simulink model "Power_Model_Official_Pars_2022a"  (R2022a)
settings: Solver=ode23t  StartTime=0.0  StopTime=500  RelTol=1e-3
values from neighbouring files (symbols this model uses):
  anode_tube_D = 0.01    [fuel_cell_battery_par.mat]
  cathode_tube_D = 0.05    [fuel_cell_battery_par.mat]
  comp_rpm_TLU = [0 1800 3600]    [fuel_cell_battery_par.mat]
  coolant_num_layers = 20    [fuel_cell_battery_par.mat]
  coolant_num_passes = 12    [fuel_cell_battery_par.mat]
  coolant_tube_D = 0.05    [fuel_cell_battery_par.mat]
  coolant_w_channels = 1    [fuel_cell_battery_par.mat]
  env_p = 0.101325    [fuel_cell_battery_par.mat]
  env_T = 20    [fuel_cell_battery_par.mat]
  env_yH20 = 0.0115436377169    [fuel_cell_battery_par.mat]
  env_yO2 = 0.21    [fuel_cell_battery_par.mat]
  radiator_air_area_fins = 11.5625    [fuel_cell_battery_par.mat]
  radiator_air_area_primary = 1.223125    [fuel_cell_battery_par.mat]
  radiator_eta_fin = 0.7    [fuel_cell_battery_par.mat]
  radiator_N_tubes = 25    [fuel_cell_battery_par.mat]
  radiator_rho = 2700    [fuel_cell_battery_par.mat]
  radiator_t_wall = 0.0001    [fuel_cell_battery_par.mat]
  radiator_tube_H = 0.0015    [fuel_cell_battery_par.mat]
  radiator_W = 0.025    [fuel_cell_battery_par.mat]
  stack_area = 280    [fuel_cell_battery_par.mat]
  stack_iL = 1.4    [fuel_cell_battery_par.mat]
  stack_mea_rho = 1800    [fuel_cell_battery_par.mat]
  stack_num_cells = 400    [fuel_cell_battery_par.mat]
  stack_num_channels = 8    [fuel_cell_battery_par.mat]
  stack_t_gdl = 250    [fuel_cell_battery_par.mat]
  stack_t_membrane = 125    [fuel_cell_battery_par.mat]
  stack_w_channels = 1    [fuel_cell_battery_par.mat]
undefined symbols (not defined in the file or in its folder): Bat, BattCapInit, BattChargeMax, BattTempBp, CapLUTBp, CapSOCBp, Em, f_fc_auxpower, f_fc_currcmd_bpt, f_fc_h2flow, f_fc_heatflow, f_fc_tmpcmd_bpt, f_fc_voltage, Mot, Np, Ns, RInt, Tc_Batt
libraries: fl_lib x89, nesl_utility x39, FuelCell_lib x32, ee_lib x3, slpidlib x3, batteryecm_lib x1, simulink_extras x1, autolibshared x1, simulink x1
(part 3 of 4)

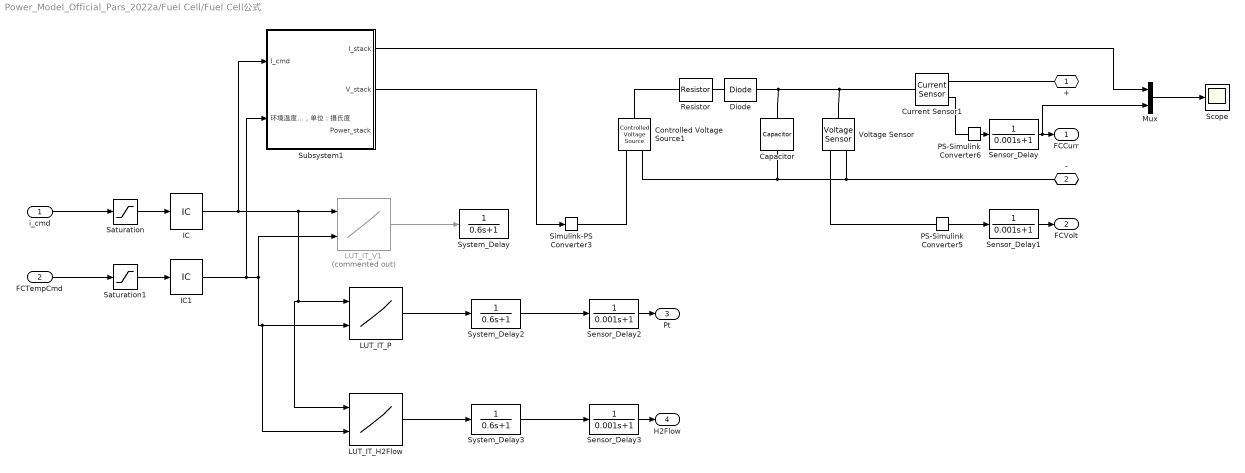
== system Power_Model_Official_Pars_2022a/Fuel Cell/Fuel Cell/公式 ==
  i_cmd : Inport
  FCTempCmd : Inport  Port=2
  Capacitor : fl_lib/Electrical/Electrical Elements/Capacitor  c=1e-6 F  r=1e-6 Ohm  g=0 1/Ohm  i_specify=off  i_priority=None  i=0 A  i_nominal_specify=off  i_nominal_unit=A  i_nominal_value=1  v_specify=off  v_priority=None  v=0 V  v_nominal_specify=off  v_nominal_unit=V  v_nominal_value=1  vc_specify=on  vc_priority=High  vc=f_fc_voltage(1) V  vc_nominal_specify=off  vc_nominal_unit=V  vc_nominal_value=1
  Controlled Voltage Source1 : fl_lib/Electrical/Electrical Sources/Controlled Voltage Source
  Current Sensor1 : fl_lib/Electrical/Electrical Sensors/Current Sensor
  Diode : fl_lib/Electrical/Electrical Elements/Diode  Vf=0.6 V  Ron=0.3 Ohm  Goff=1e-8 1/Ohm  i_specify=off  i_priority=None  i=0 A  i_nominal_specify=off  i_nominal_unit=A  i_nominal_value=1  v_specify=off  v_priority=None  v=0 V  v_nominal_specify=off  v_nominal_unit=V  v_nominal_value=1
  IC : InitialCondition  Value=f_fc_currcmd_bpt(1)
  IC1 : InitialCondition  Value=f_fc_tmpcmd_bpt(1)
  LUT_IT_H2Flow : Lookup_n-D  BreakpointsForDimension1=f_fc_currcmd_bpt  BreakpointsForDimension2=f_fc_tmpcmd_bpt  Table=f_fc_h2flow  InternalRulePriority=Speed  RndMeth=Simplest
      settings: InputPortMap=u0,u1
  LUT_IT_P : Lookup_n-D  BreakpointsForDimension1=f_fc_currcmd_bpt  BreakpointsForDimension2=f_fc_tmpcmd_bpt  Table=f_fc_auxpower  InternalRulePriority=Speed  RndMeth=Simplest
      settings: InputPortMap=u0,u1
  LUT_IT_V1 : Lookup_n-D  Commented=on  BreakpointsForDimension1=f_fc_currcmd_bpt  BreakpointsForDimension2=f_fc_tmpcmd_bpt  Table=f_fc_voltage  InternalRulePriority=Speed  RndMeth=Simplest
      settings: InputPortMap=u0,u1
  Mux : Mux  Inputs=2
  PS-Simulink Converter5 : nesl_utility/PS-Simulink Converter  PhysicalDomain=network_engine_domain  SubClassName=ps_output  LeftPortType=input  RightPortType=output  PseudoPeriodic=off  Frequencies=[]  VectorFormat=1-D array  Unit=inherit  AffineConversion=off
  PS-Simulink Converter6 : nesl_utility/PS-Simulink Converter  PhysicalDomain=network_engine_domain  SubClassName=ps_output  LeftPortType=input  RightPortType=output  PseudoPeriodic=off  Frequencies=[]  VectorFormat=1-D array  Unit=1  AffineConversion=off
  Resistor : fl_lib/Electrical/Electrical Elements/Resistor  R=1e-3 Ohm  i_specify=off  i_priority=None  i=0 A  i_nominal_specify=off  i_nominal_unit=A  i_nominal_value=1  v_specify=off  v_priority=None  v=0 V  v_nominal_specify=off  v_nominal_unit=V  v_nominal_value=1
  Saturation : Saturate  UpperLimit=max(f_fc_currcmd_bpt)  LowerLimit=0
  Saturation1 : Saturate  UpperLimit=max(f_fc_tmpcmd_bpt)  LowerLimit=0
  Scope : Scope
  Sensor_Delay{,1..3} (4 alike) : TransferFcn  Denominator=[0.001 1]
  Simulink-PS Converter3 : nesl_utility/Simulink-PS Converter  PhysicalDomain=network_engine_domain  SubClassName=ps_input  LeftPortType=input  RightPortType=output  PseudoPeriodic=off  Frequencies=[]  NoiseDistribution=none  NoiseParameters=[]  Unit=V  AffineConversion=off  FilteringAndDerivatives=provide  SimscapeFilterOrder=1  InputFilterTimeConstant=0.001  UdotUserProvided=0
  Subsystem1 : Subsystem
  System_Delay : TransferFcn  Denominator=[0.6 1]
  System_Delay2 : TransferFcn  Denominator=[0.6 1]
  System_Delay3 : TransferFcn  Denominator=[0.6 1]
  Voltage Sensor : fl_lib/Electrical/Electrical Sensors/Voltage Sensor
  + : PMIOPort  Side=Right
  - : PMIOPort  Port=2  Side=Right
  FCCurr : Outport
  FCVolt : Outport  Port=2
  Pt : Outport  Port=3
  H2Flow : Outport  Port=4
  wires:
  LUT_IT_H2Flow/1 -> System_Delay3/1
  System_Delay3/1 -> Sensor_Delay3/1
  Saturation1/1 -> IC1/1
  LUT_IT_V1/1 -> System_Delay/1
  Sensor_Delay/1 -> Mux/2, FCCurr/1
  IC1/1 -> Subsystem1/2(环境温度：T，单位：摄氏度), LUT_IT_V1/2, LUT_IT_H2Flow/2, LUT_IT_P/2
  Saturation/1 -> IC/1
  LUT_IT_P/1 -> System_Delay2/1
  IC/1 -> Subsystem1/1(I_cmd), LUT_IT_H2Flow/1, LUT_IT_P/1, LUT_IT_V1/1
  FCTempCmd/1 -> Saturation1/1
  i_cmd/1 -> Saturation/1
  Sensor_Delay2/1 -> Pt/1
  Sensor_Delay3/1 -> H2Flow/1
  PS-Simulink Converter5/1 -> Sensor_Delay1/1
  Sensor_Delay1/1 -> FCVolt/1
  PS-Simulink Converter6/1 -> Sensor_Delay/1
  Subsystem1/2(V_stack) -> Simulink-PS Converter3/1
  System_Delay2/1 -> Sensor_Delay2/1
  Subsystem1/1(I_stack) -> Mux/1
  Mux/1 -> Scope/1
  connections:
  Capacitor/RConn1 -- Voltage Sensor/RConn2 -- -/RConn1 -- Controlled Voltage Source1/RConn2
  Capacitor/LConn1 -- Diode/RConn1 -- Voltage Sensor/LConn1 -- Current Sensor1/LConn1
  +/RConn1 -- Current Sensor1/RConn2
  PS-Simulink Converter5/LConn1 -- Voltage Sensor/RConn1
  PS-Simulink Converter6/LConn1 -- Current Sensor1/RConn1
  Simulink-PS Converter3/RConn1 -- Controlled Voltage Source1/RConn1
  Resistor/RConn1 -- Diode/LConn1
  Resistor/LConn1 -- Controlled Voltage Source1/LConn1

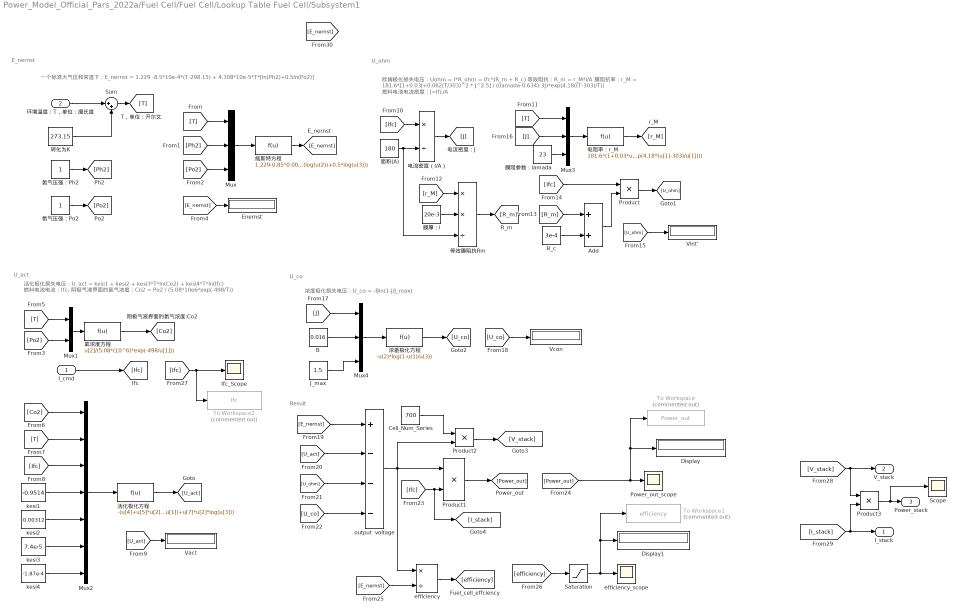
== system Power_Model_Official_Pars_2022a/Fuel Cell/Fuel Cell/Lookup Table Fuel Cell/Subsystem1 ==
  note: Result
  note: U_co
  note: 浓度极化损失电压：U_co = -Bln(1-J/J_max)
  note: U_ohm
  note: 欧姆极化损失电压：Uohm = I*R_ohm = Ifc*(R_m + R_c)
      | 等效阻抗：R_m = r_M*l/A
      | 膜阻抗率：r_M = 181.6*[1+0.03J+0.062(T/303)^2 * J^2.5] / ((lamada-0.634)-3J)*exp(4.18((T-303)/T))
      | 燃料电池电流密度：J=Ifc/A
  note: U_act
  note: 活化极化损失电压：U_act = kesi1 + kesi2 + kesi3*T*ln(Co2) + kesi4*T*ln(Ifc)
      | 燃料电池电流：Ifc;
      | 阴极气液界面的氧气浓度：Co2 = Po2 / (5.08*10e6*exp(-498/T))
  note: E_nernst
  note: 一个标准大气压和常温下：E_nernst = 1.229 -8.5*10e-4*(T-298.15) + 4.308*10e-5*T*[ln(Ph2)+0.5ln(Po2)]
  I_cmd : Inport
  环境温度：T，单位：摄氏度 : Inport  Port=2
  Add : Sum
  B : Constant  Value=0.016
  Cell_Num_Series : Constant  Value=700
  Display : Display
  Display1 : Display
  Enernst : Display
      settings: Decimation=5
  Ifc_Scope : Scope
  J_max : Constant  Value=1.5
  Mux : Mux  Inputs=3
  Mux1 : Mux  Inputs=2
  Mux2 : Mux  Inputs=7
  Mux3 : Mux  Inputs=3
  Mux4 : Mux  Inputs=3
  Power_out_scope : Scope
  Product{,1..3} (4 alike) : Product
  R_c : Constant  Value=3e-4
  Saturation : Saturate  UpperLimit=0.9  LowerLimit=0
  Scope : Scope
  Sum : Sum  Inputs=|++
  To Workspace : ToWorkspace  Commented=on  VariableName=Power_out  SampleTime=-1
      settings: Save2DSignal=2-D array (concatenate along first dimension)
  To Workspace1 : ToWorkspace  Commented=on  VariableName=efficiency  SampleTime=-1
      settings: Save2DSignal=2-D array (concatenate along first dimension)
  To Workspace2 : ToWorkspace  Commented=on  VariableName=Ifc  SampleTime=-1
      settings: Save2DSignal=2-D array (concatenate along first dimension)
  Vact : Display
      settings: Decimation=5
  Vcon : Display
      settings: Decimation=5
  Vint' : Display
      settings: Decimation=5
  efficiency : Product  Inputs=*/  OutDataTypeStr=double
  efficiency_scope : Scope
  kesi1 : Constant  Value=-0.9514
  kesi2 : Constant  Value=0.00312
  kesi3 : Constant  Value=7.4e-5
  kesi4 : Constant  Value=-1.87e-4
  output  voltage : Sum  Inputs=+---  OutDataTypeStr=double
  氢气压强：Ph2 : Constant
  氧气压强：Po2 : Constant
  氧浓度方程 : Fcn  Expr=u[2]/(5.08*(10^6)*exp(-498/u[1]))
  活化极化方程 : Fcn  Expr=-(u[4]+u[5]*u[2]+u[6]*u[2]*log(u[1])+u[7]*u[2]*log(u[3]))
  浓差极化方程 : Fcn  Expr=-u(2)*log(1-u(1)/u(3))
  电流密度（I/A） : Product  Inputs=*/  OutDataTypeStr=double
  电阻率：r_M : Fcn  Expr=181.6*(1+0.03*u[2]+0.062*((u[1]/303)^2)*(u[2]^2.5))/((u[3]-0.634-3*u[2])*(exp(4.18*(u[1]-303)/u[1])))
  等效膜阻抗Rm : Product  Inputs=**/  OutDataTypeStr=double
  能斯特方程 : Fcn  Expr=1.229-0.85*0.001*(u(1)-298.15)+4.3085*0.00001*u(1)*(log(u(2))+0.5*log(u(3)))
  膜厚：l : Constant  Value=20e-3
  膜阻参数：lamada : Constant  Value=23
  转化为K : Constant  Value=273.15
  面积(A) : Constant  Value=180
  I_stack : Outport
  V_stack : Outport  Port=2
  Power_stack : Outport  Port=3
  wires:
  [E_nernst] -> efficiency/2
  环境温度：T，单位：摄氏度/1 -> Sum/1
  [T] -> Mux/1
  Sum/1 -> [T]
  [Ifc] -> 电流密度（I/A）/1
  [Co2] -> Mux2/1
  Mux2/1 -> 活化极化方程/1
  [T] -> Mux2/2
  转化为K/1 -> Sum/2
  能斯特方程/1 -> [E_nernst]
  [Ifc] -> To Workspace2/1, Ifc_Scope/1
  Saturation/1 -> efficiency_scope/1, To Workspace1/1, Display1/1
  面积(A)/1 -> 电流密度（I/A）/2, 等效膜阻抗Rm/3
  [T] -> Mux1/1
  活化极化方程/1 -> [U_act]
  电流密度（I/A）/1 -> [J]
  output  voltage/1 -> Product2/2, efficiency/1, Product1/1
  [U_act] -> output  voltage/2
  氧气压强：Po2/1 -> [Po2]
  [r_M] -> 等效膜阻抗Rm/1
  氢气压强：Ph2/1 -> [Ph2]
  [Ifc] -> Product/1
  等效膜阻抗Rm/1 -> [R_m]
  efficiency/1 -> [efficiency]
  R_c/1 -> Add/2
  Mux4/1 -> 浓差极化方程/1
  [E_nernst] -> Enernst/1
  [Ph2] -> Mux/2
  kesi2/1 -> Mux2/5
  J_max/1 -> Mux4/3
  膜厚：l/1 -> 等效膜阻抗Rm/2
  [efficiency] -> Saturation/1
  [R_m] -> Add/1
  [U_co] -> Vcon/1
  [Power_out] -> Power_out_scope/1, To Workspace/1, Display/1
  Product1/1 -> [Power_out]
  [J] -> Mux4/1
  [U_ohm] -> output  voltage/3
  Cell_Num_Series/1 -> Product2/1
  浓差极化方程/1 -> [U_co]
  [V_stack] -> V_stack/1, Product3/1
  kesi1/1 -> Mux2/4
  kesi4/1 -> Mux2/7
  [U_act] -> Vact/1
  Mux1/1 -> 氧浓度方程/1
  Mux/1 -> 能斯特方程/1
  [Po2] -> Mux1/2
  膜阻参数：lamada/1 -> Mux3/3
  [Po2] -> Mux/3
  kesi3/1 -> Mux2/6
  [I_stack] -> I_stack/1, Product3/2
  [U_ohm] -> Vint'/1
  氧浓度方程/1 -> [Co2]
  B/1 -> Mux4/2
  Mux3/1 -> 电阻率：r_M/1
  [T] -> Mux3/1
  电阻率：r_M/1 -> [r_M]
  Add/1 -> Product/2
  [E_nernst] -> output  voltage/1
  [Ifc] -> Mux2/3
  [Ifc] -> [I_stack], Product1/2
  [J] -> Mux3/2
  [U_co] -> output  voltage/4
  Product/1 -> [U_ohm]
  Product3/1 -> Scope/1, Power_stack/1
  I_cmd/1 -> [Ifc]
  Product2/1 -> [V_stack]

== system Power_Model_Official_Pars_2022a/Fuel Cell/Fuel Cell/Simscape Fuel Cell_2/Anode Humidifier ==
  Composition and Humidity Sensor (FC) : FuelCell_lib/sensors/Composition and Humidity Sensor (FC)
      settings: InternalSimscapePortConfiguration="{\"Bottom\":[],\"Left\":[{\"id\":\"A\",\"label\":\"A\",\"type\":\"FuelCell.FuelCell\"}],\"Right\":[{\"id\":\"x_i\",\"label\":\"x_i\",\"type\":\"output\"},{\"id\":\"y_i\",\"label\":\"y_i\",\"type\":\"output\"},{\"id\":\"W\",\"label\":\"W\",\"type\":\"output\"}],\"Top\":[]}"
  PS Gain : fl_lib/Physical Signals/Functions/PS Gain  gain=[0;0;0;1]
  PS-Simulink Converter : nesl_utility/PS-Simulink Converter  PhysicalDomain=network_engine_domain  SubClassName=ps_output  LeftPortType=input  RightPortType=output  PseudoPeriodic=off  Frequencies=[]  VectorFormat=1-D array  Unit=1  AffineConversion=off
  Perfect Insulator : fl_lib/Thermal/Thermal Elements/Perfect Insulator  T_specify=off  T_priority=None  T=0 K  T_nominal_specify=off  T_nominal_unit=K  T_nominal_value=1
  Pipe (N Gas) : FuelCell_lib/elements/Pipe (FC)  length=0.25 m  area=pi*0.05^2/4 m^2  Dh=0.05 m  extra_length=0.1 m  roughness=15e-6 m  Re_lam=2000  Re_tur=4000  shape_factor=64  Nu_lam=3.66  tau_c=1e-3 s  isCond=[0; 0; 0; 0]  volMeas=false  compMeas=FuelCell.enum.Composition.Mole  p0=env_p MPa  T0=env_T degC  comp=FuelCell.enum.Composition.Mole  y0=[0; 0; 1; 0]  x0=[1; 0; 0; 0]
      settings: InternalSimscapePortConfiguration="{\"Bottom\":[{\"id\":\"MIn\",\"label\":\"M_in\",\"type\":\"input\"},{\"id\":\"TIn\",\"label\":\"T_in\",\"type\":\"input\"}],\"Left\":[{\"id\":\"A\",\"label\":\"A\",\"type\":\"FuelCell.FuelCell\"},{\"id\":\"H\",\"label\":\"H\",\"type\":\"foundation.thermal.thermal\"}],\"Right\":[{\"id\":\"B\",\"label\":\"B\",\"type\":\"FuelCell.FuelCell\"}],\"Top\":[]}"
  Proportional Control : Subsystem
  Relative Humidity : Constant
  Simulink-PS Converter : nesl_utility/Simulink-PS Converter  PhysicalDomain=network_engine_domain  SubClassName=ps_input  LeftPortType=input  RightPortType=output  PseudoPeriodic=off  Frequencies=[]  NoiseDistribution=none  NoiseParameters=[]  Unit=kg/s  AffineConversion=off  FilteringAndDerivatives=provide  SimscapeFilterOrder=1  InputFilterTimeConstant=0.001  UdotUserProvided=0
  Simulink-PS Converter1 : nesl_utility/Simulink-PS Converter  PhysicalDomain=network_engine_domain  SubClassName=ps_input  LeftPortType=input  RightPortType=output  PseudoPeriodic=off  Frequencies=[]  NoiseDistribution=none  NoiseParameters=[]  Unit=degC  AffineConversion=on  FilteringAndDerivatives=provide  SimscapeFilterOrder=1  InputFilterTimeConstant=0.001  UdotUserProvided=0
  Transfer Fcn : TransferFcn  Denominator=[1 1]
  A : PMIOPort  Side=Left
  B : PMIOPort  Port=2  Side=Right
  wires:
  Transfer Fcn/1 -> Simulink-PS Converter1/1
  [T_stack] -> Transfer Fcn/1
  Relative Humidity/1 -> Proportional Control/1(RH_set)
  PS-Simulink Converter/1 -> Proportional Control/2(RH_meas)
  Proportional Control/1(Mw) -> Simulink-PS Converter/1
  connections:
  PS Gain/LConn1 -- Simulink-PS Converter/RConn1
  Simulink-PS Converter1/RConn1 -- Pipe (N Gas)/RConn3
  PS-Simulink Converter/LConn1 -- Composition and Humidity Sensor (FC)/RConn3
  Pipe (N Gas)/RConn1 -- Composition and Humidity Sensor (FC)/LConn1 -- B/RConn1
  A/RConn1 -- Pipe (N Gas)/LConn1
  Perfect Insulator/LConn1 -- Pipe (N Gas)/LConn2
  PS Gain/RConn1 -- Pipe (N Gas)/RConn2

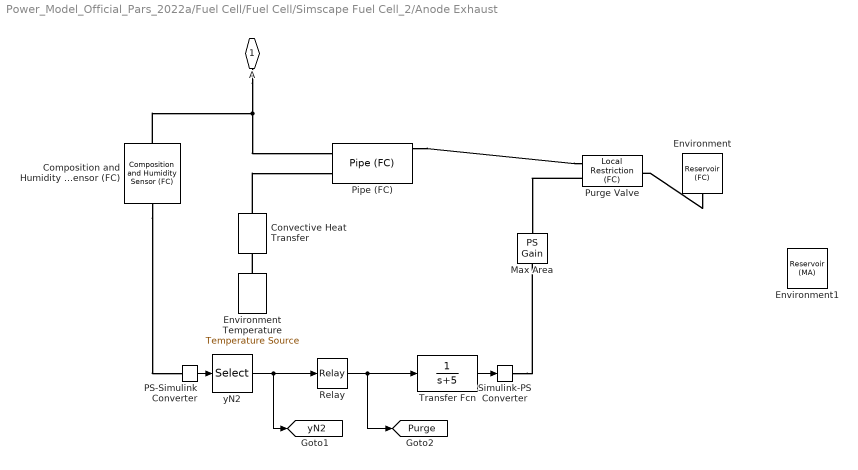
== system Power_Model_Official_Pars_2022a/Fuel Cell/Fuel Cell/Simscape Fuel Cell_2/Anode Exhaust ==
  Composition and Humidity Sensor (FC) : FuelCell_lib/sensors/Composition and Humidity Sensor (FC)
      settings: InternalSimscapePortConfiguration="{\"Bottom\":[],\"Left\":[{\"id\":\"A\",\"label\":\"A\",\"type\":\"FuelCell.FuelCell\"}],\"Right\":[{\"id\":\"x_i\",\"label\":\"x_i\",\"type\":\"output\"},{\"id\":\"y_i\",\"label\":\"y_i\",\"type\":\"output\"},{\"id\":\"W\",\"label\":\"W\",\"type\":\"output\"}],\"Top\":[]}"
  Convective Heat Transfer : fl_lib/Thermal/Thermal Elements/Convective Heat Transfer  thermal_type=foundation.enum.constant_variable.constant  area=pi*anode_tube_D^2/4 m^2  heat_tr_coeff=20 W/(m^2 * K)  min_heat_tr_coeff=1e-3 W/(K*m^2)  T_specify=off  T_priority=None  T=0 K  T_nominal_specify=off  T_nominal_unit=K  T_nominal_value=1  Q_specify=off  Q_priority=None  Q=0 W  Q_nominal_specify=off  Q_nominal_unit=W  Q_nominal_value=1
  Environment : FuelCell_lib/elements/Reservoir (FC)  constCond=true  p0=env_p MPa  T0=env_T degC  comp=FuelCell.enum.Composition.Mole  y0=[1-env_yO2-env_yH20; env_yO2; 0; env_yH20]  x0=[1; 0; 0; 0]  area=pi*anode_tube_D^2/4 m^2
      settings: InternalSimscapePortConfiguration="{\"Bottom\":[],\"Left\":[],\"Right\":[],\"Top\":[{\"id\":\"A\",\"label\":\"A\",\"type\":\"FuelCell.FuelCell\"}]}"
  Environment Temperature : fl_lib/Thermal/Thermal Sources/Temperature Source  temperature=env_T degC
  Environment1 : fl_lib/Moist Air/Elements/Reservoir (MA)  pressure_spec=foundation.enum.pressure_spec.specified  reservoir_pressure=env_p MPa  temperature_spec=foundation.enum.temperature_spec.specified  reservoir_temperature=env_T degC  moisture_spec=foundation.enum.moisture_spec.relative_humidity  reservoir_RH=0  reservoir_x_w=0.01  reservoir_y_w=0.01  reservoir_HR=0.01  reservoir_Tw=287 K  trace_gas_spec=foundation.enum.trace_gas_spec.mole_fraction  reservoir_x_g=0.001  reservoir_y_g=tank_yH2  RH_ws=1  area_A=pi*anode_tube_D^2/4 m^2
  Max Area : fl_lib/Physical Signals/Functions/PS Gain  gain=pi*(anode_tube_D)^2/4 m^2
  PS-Simulink Converter : nesl_utility/PS-Simulink Converter  PhysicalDomain=network_engine_domain  SubClassName=ps_output  LeftPortType=input  RightPortType=output  PseudoPeriodic=off  Frequencies=[]  VectorFormat=inherit  Unit=inherit  AffineConversion=off
  Pipe (FC) : FuelCell_lib/elements/Pipe (FC)  length=1 m  area=pi*anode_tube_D^2/4 m^2  Dh=anode_tube_D m  extra_length=0.1 m  roughness=15e-6 m  Re_lam=2000  Re_tur=4000  shape_factor=64  Nu_lam=3.66  tau_c=1e-3 s  isCond=[0; 0; 0; 0]  volMeas=false  compMeas=FuelCell.enum.Composition.Mole  p0=env_p MPa  T0=env_T degC  comp=FuelCell.enum.Composition.Mole  y0=[0; 0; 1; 0]  x0=[1; 0; 0; 0]
      settings: InternalSimscapePortConfiguration="{\"Bottom\":[{\"id\":\"MIn\",\"label\":\"M_in\",\"type\":\"input\"},{\"id\":\"TIn\",\"label\":\"T_in\",\"type\":\"input\"}],\"Left\":[{\"id\":\"A\",\"label\":\"A\",\"type\":\"FuelCell.FuelCell\"},{\"id\":\"H\",\"label\":\"H\",\"type\":\"foundation.thermal.thermal\"}],\"Right\":[{\"id\":\"B\",\"label\":\"B\",\"type\":\"FuelCell.FuelCell\"}],\"Top\":[]}"
  Purge Valve : FuelCell_lib/elements/Local Restriction (FC)  const_area=false  restriction_area=0.001 m^2  min_area=pi*(1e-4*anode_tube_D)^2/4 m^2  max_area=pi*(0.5*anode_tube_D)^2/4 m^2  area=pi*anode_tube_D^2/4 m^2  Cd=0.64  B_lam=0.999
      settings: InternalSimscapePortConfiguration="{\"Bottom\":[],\"Left\":[{\"id\":\"AR\",\"label\":\"AR\",\"type\":\"input\"},{\"id\":\"A\",\"label\":\"A\",\"type\":\"FuelCell.FuelCell\"}],\"Right\":[{\"id\":\"B\",\"label\":\"B\",\"type\":\"FuelCell.FuelCell\"}],\"Top\":[]}"
  Relay : Relay  OnSwitchValue=0.5  OffSwitchValue=0.1
  Simulink-PS Converter : nesl_utility/Simulink-PS Converter  PhysicalDomain=network_engine_domain  SubClassName=ps_input  LeftPortType=input  RightPortType=output  PseudoPeriodic=off  Frequencies=[]  NoiseDistribution=none  NoiseParameters=[]  Unit=1  AffineConversion=off  FilteringAndDerivatives=provide  SimscapeFilterOrder=1  InputFilterTimeConstant=0.001  UdotUserProvided=0
  Transfer Fcn : TransferFcn  Denominator=[1 5]
  yN2 : Selector  InputPortWidth=4  IndexOptions=Index vector (dialog)  Indices=1  OutputSizes=1
  A : PMIOPort  Side=Left
  tag scope: Purge=global, yN2=global
  wires:
  Relay/1 -> [Purge], Transfer Fcn/1
  Transfer Fcn/1 -> Simulink-PS Converter/1
  yN2/1 -> [yN2], Relay/1
  PS-Simulink Converter/1 -> yN2/1
  connections:
  A/RConn1 -- Composition and Humidity Sensor (FC)/LConn1 -- Pipe (FC)/LConn1
  Simulink-PS Converter/RConn1 -- Max Area/LConn1
  Purge Valve/LConn1 -- Max Area/RConn1
  Convective Heat Transfer/LConn1 -- Pipe (FC)/LConn2
  Environment Temperature/LConn1 -- Convective Heat Transfer/RConn1
  Pipe (FC)/RConn1 -- Purge Valve/LConn2
  Environment/LConn1 -- Purge Valve/RConn1
  Composition and Humidity Sensor (FC)/RConn2 -- PS-Simulink Converter/LConn1

== system Power_Model_Official_Pars_2022a/Fuel Cell/Fuel Cell/Simscape Fuel Cell_2/Anode Gas Channels ==
  Anode : FuelCell_lib/elements/Constant Volume Chamber (FC)  V0=stack_w_channels^2 * stack_num_channels * stack_num_cells * sqrt(stack_area) cm^3  num_ports=foundation.enum.num_ports.three  area_A=stack_w_channels^2 * stack_num_channels * stack_num_cells cm^2  area_B=stack_w_channels^2 * stack_num_channels * stack_num_cells cm^2  area_C=stack_w_channels^2 * stack_num_channels * stack_num_cells cm^2  area_D=0.01 m^2  cond_spec=FuelCell.enum.ChamberCondSpec.Enabled  tau_c=1e-3 s  is_cond=[0; 0; 0; 0]  out_comp=FuelCell.enum.Composition.Mass  p0=env_p MPa  T0=env_T degC  comp=FuelCell.enum.Composition.Mole  y0=[0; 0; 1; 0]  x0=[1; 0; 0; 0]
      settings: InternalSimscapePortConfiguration="{\"Bottom\":[{\"id\":\"H\",\"label\":\"H\",\"type\":\"foundation.thermal.thermal\"}],\"Left\":[{\"id\":\"MIn\",\"label\":\"MIn\",\"type\":\"input\"},{\"id\":\"TIn\",\"label\":\"TIn\",\"type\":\"input\"}],\"Right\":[{\"id\":\"pC\",\"label\":\"p\",\"type\":\"output\"},{\"id\":\"TC\",\"label\":\"T\",\"type\":\"output\"},{\"id\":\"xC_i\",\"label\":\"x_i\",\"type\":\"output\"}],\"Top\":[{\"id\":\"A\",\"label\":\"A\",\"type\":\"FuelCell.FuelCell\"},{\"id\":\"B\",\"label\":\"B\",\"type\":\"FuelCell.FuelCell\"},{\"id\":\"C\",\"label\":\"C\",\"type\":\"FuelCell.FuelCell\"}]}"
  A : PMIOPort  Side=Right
  Min : PMIOPort  Port=2  Side=Right
  Tin : PMIOPort  Port=3  Side=Right
  H : PMIOPort  Port=4  Side=Right
  B : PMIOPort  Port=5  Side=Left
  C : PMIOPort  Port=6  Side=Left
  xi : PMIOPort  Port=7  Side=Left
  connections:
  B/RConn1 -- Anode/LConn4
  Min/RConn1 -- Anode/LConn1
  Tin/RConn1 -- Anode/LConn2
  xi/RConn1 -- Anode/RConn3
  Anode/LConn5 -- C/RConn1
  A/RConn1 -- Anode/LConn3
  H/RConn1 -- Anode/RConn4

== system Power_Model_Official_Pars_2022a/Fuel Cell/Fuel Cell/Simscape Fuel Cell_2/Cathode Humidifier ==
  Composition and Humidity Sensor (FC) : FuelCell_lib/sensors/Composition and Humidity Sensor (FC)
      settings: InternalSimscapePortConfiguration="{\"Bottom\":[],\"Left\":[{\"id\":\"A\",\"label\":\"A\",\"type\":\"FuelCell.FuelCell\"}],\"Right\":[{\"id\":\"x_i\",\"label\":\"x_i\",\"type\":\"output\"},{\"id\":\"y_i\",\"label\":\"y_i\",\"type\":\"output\"},{\"id\":\"W\",\"label\":\"W\",\"type\":\"output\"}],\"Top\":[]}"
  PS Gain1 : fl_lib/Physical Signals/Functions/PS Gain  gain=[0;0;0;1]
  PS-Simulink Converter2 : nesl_utility/PS-Simulink Converter  PhysicalDomain=network_engine_domain  SubClassName=ps_output  LeftPortType=input  RightPortType=output  PseudoPeriodic=off  Frequencies=[]  VectorFormat=1-D array  Unit=1  AffineConversion=off
  Perfect Insulator : fl_lib/Thermal/Thermal Elements/Perfect Insulator  T_specify=off  T_priority=None  T=0 K  T_nominal_specify=off  T_nominal_unit=K  T_nominal_value=1
  Pipe (FC) : FuelCell_lib/elements/Pipe (FC)  length=0.25 m  area=pi*0.05^2/4 m^2  Dh=0.05 m  extra_length=0.1 m  roughness=15e-6 m  Re_lam=2000  Re_tur=4000  shape_factor=64  Nu_lam=3.66  tau_c=1e-3 s  isCond=[0; 0; 0; 0]  volMeas=false  compMeas=FuelCell.enum.Composition.Mole  p0=env_p MPa  T0=env_T degC  comp=FuelCell.enum.Composition.Mole  y0=[1-env_yO2-env_yH20; env_yO2; 0; env_yH20]  x0=[1; 0; 0; 0]
      settings: InternalSimscapePortConfiguration="{\"Bottom\":[{\"id\":\"MIn\",\"label\":\"M_in\",\"type\":\"input\"},{\"id\":\"TIn\",\"label\":\"T_in\",\"type\":\"input\"}],\"Left\":[{\"id\":\"A\",\"label\":\"A\",\"type\":\"FuelCell.FuelCell\"},{\"id\":\"H\",\"label\":\"H\",\"type\":\"foundation.thermal.thermal\"}],\"Right\":[{\"id\":\"B\",\"label\":\"B\",\"type\":\"FuelCell.FuelCell\"}],\"Top\":[]}"
  Proportional Control : Subsystem
  Relative Humidity : Constant
  Simulink-PS Converter2 : nesl_utility/Simulink-PS Converter  PhysicalDomain=network_engine_domain  SubClassName=ps_input  LeftPortType=input  RightPortType=output  PseudoPeriodic=off  Frequencies=[]  NoiseDistribution=none  NoiseParameters=[]  Unit=kg/s  AffineConversion=off  FilteringAndDerivatives=provide  SimscapeFilterOrder=1  InputFilterTimeConstant=0.001  UdotUserProvided=0
  Simulink-PS Converter3 : nesl_utility/Simulink-PS Converter  PhysicalDomain=network_engine_domain  SubClassName=ps_input  LeftPortType=input  RightPortType=output  PseudoPeriodic=off  Frequencies=[]  NoiseDistribution=none  NoiseParameters=[]  Unit=degC  AffineConversion=on  FilteringAndDerivatives=provide  SimscapeFilterOrder=1  InputFilterTimeConstant=0.001  UdotUserProvided=0
  Transfer Fcn1 : TransferFcn  Denominator=[1 1]
  A : PMIOPort  Side=Right
  B : PMIOPort  Port=2  Side=Left
  wires:
  Transfer Fcn1/1 -> Simulink-PS Converter3/1
  [T_stack] -> Transfer Fcn1/1
  Relative Humidity/1 -> Proportional Control/1(RH_set)
  PS-Simulink Converter2/1 -> Proportional Control/2(RH_meas)
  Proportional Control/1(Mw) -> Simulink-PS Converter2/1
  connections:
  A/RConn1 -- Pipe (FC)/LConn1
  Simulink-PS Converter3/RConn1 -- Pipe (FC)/RConn3
  Pipe (FC)/LConn2 -- Perfect Insulator/LConn1
  B/RConn1 -- Composition and Humidity Sensor (FC)/LConn1 -- Pipe (FC)/RConn1
  PS Gain1/RConn1 -- Pipe (FC)/RConn2
  Simulink-PS Converter2/RConn1 -- PS Gain1/LConn1
  PS-Simulink Converter2/LConn1 -- Composition and Humidity Sensor (FC)/RConn3

== system Power_Model_Official_Pars_2022a/Fuel Cell/Fuel Cell/Simscape Fuel Cell_2/Cathode Exhaust ==
  Constant1 : Constant  Value=env_p
  Convective Heat Transfer1 : fl_lib/Thermal/Thermal Elements/Convective Heat Transfer  thermal_type=foundation.enum.constant_variable.constant  area=pi*cathode_tube_D*1 m^2  heat_tr_coeff=20 W/(m^2 * K)  min_heat_tr_coeff=1e-3 W/(K*m^2)  T_specify=off  T_priority=None  T=0 K  T_nominal_specify=off  T_nominal_unit=K  T_nominal_value=1  Q_specify=off  Q_priority=None  Q=0 W  Q_nominal_specify=off  Q_nominal_unit=W  Q_nominal_value=1
  Environment : FuelCell_lib/elements/Reservoir (FC)  constCond=true  p0=env_p MPa  T0=env_T degC  comp=FuelCell.enum.Composition.Mole  y0=[1-env_yO2-env_yH20; env_yO2; 0; env_yH20]  x0=[1; 0; 0; 0]  area=pi*cathode_tube_D^2/4 m^2
      settings: InternalSimscapePortConfiguration="{\"Bottom\":[],\"Left\":[],\"Right\":[],\"Top\":[{\"id\":\"A\",\"label\":\"A\",\"type\":\"FuelCell.FuelCell\"}]}"
  Environment Temperature : fl_lib/Thermal/Thermal Sources/Temperature Source  temperature=env_T degC
  Pipe (N Gas)1 : FuelCell_lib/elements/Pipe (FC)  length=1 m  area=pi*cathode_tube_D^2/4 m^2  Dh=cathode_tube_D m  extra_length=0.1 m  roughness=15e-6 m  Re_lam=2000  Re_tur=4000  shape_factor=64  Nu_lam=3.66  tau_c=1e-3 s  isCond=[0; 0; 0; 0]  volMeas=false  compMeas=FuelCell.enum.Composition.Mole  p0=env_p MPa  T0=env_T degC  comp=FuelCell.enum.Composition.Mole  y0=[1-env_yO2-env_yH20; env_yO2; 0; env_yH20]  x0=[1; 0; 0; 0]
      settings: InternalSimscapePortConfiguration="{\"Bottom\":[{\"id\":\"MIn\",\"label\":\"M_in\",\"type\":\"input\"},{\"id\":\"TIn\",\"label\":\"T_in\",\"type\":\"input\"}],\"Left\":[{\"id\":\"A\",\"label\":\"A\",\"type\":\"FuelCell.FuelCell\"},{\"id\":\"H\",\"label\":\"H\",\"type\":\"foundation.thermal.thermal\"}],\"Right\":[{\"id\":\"B\",\"label\":\"B\",\"type\":\"FuelCell.FuelCell\"}],\"Top\":[]}"
  Pressure Relief Valve : Subsystem  Tag=PublishSubsystem  mask(Pressure Relief Valve){D=cathode_tube_D, r_min=1e-4, r_max=0.8, p_range=0.005}
      mask prompts: D "Connecting tube diameter (m)"; r_min "Min diameter ratio"; r_max "Max diameter ratio"; p_range "Pressure regulation range (MPa)"
      mask help: This subsystem models a pressure relief valve that maintains a set pressure at port A. The valve is normally closed. When the pressure is above the set pressure, it begins to open.
  Simulink-PS Converter1 : nesl_utility/Simulink-PS Converter  PhysicalDomain=network_engine_domain  SubClassName=ps_input  LeftPortType=input  RightPortType=output  PseudoPeriodic=off  Frequencies=[]  NoiseDistribution=none  NoiseParameters=[]  Unit=MPa  AffineConversion=off  FilteringAndDerivatives=provide  SimscapeFilterOrder=1  InputFilterTimeConstant=0.001  UdotUserProvided=0
  Stack Pressure : Constant  Value=0.06
  Sum : Sum  Inputs=++|
  C : PMIOPort  Side=Left
  wires:
  Stack Pressure/1 -> Sum/1
  Sum/1 -> Simulink-PS Converter1/1
  Constant1/1 -> Sum/2
  connections:
  C/RConn1 -- Pipe (N Gas)1/LConn1
  Simulink-PS Converter1/RConn1 -- Pressure Relief Valve/LConn2
  Pipe (N Gas)1/RConn1 -- Pressure Relief Valve/LConn1
  Pressure Relief Valve/RConn1 -- Environment/LConn1
  Convective Heat Transfer1/LConn1 -- Pipe (N Gas)1/LConn2
  Environment Temperature/LConn1 -- Convective Heat Transfer1/RConn1

== system Power_Model_Official_Pars_2022a/Fuel Cell/Fuel Cell/Simscape Fuel Cell_2/Cathode Gas Channels ==
  Cathode : FuelCell_lib/elements/Constant Volume Chamber (FC)  V0=stack_w_channels^2 * stack_num_channels * stack_num_cells * sqrt(stack_area) cm^3  num_ports=foundation.enum.num_ports.three  area_A=stack_w_channels^2 * stack_num_channels * stack_num_cells cm^2  area_B=stack_w_channels^2 * stack_num_channels * stack_num_cells cm^2  area_C=stack_w_channels^2 * stack_num_channels * stack_num_cells cm^2  area_D=0.01 m^2  cond_spec=FuelCell.enum.ChamberCondSpec.Enabled  tau_c=1e-3 s  is_cond=[0; 0; 0; 0]  out_comp=FuelCell.enum.Composition.Mass  p0=env_p MPa  T0=env_T degC  comp=FuelCell.enum.Composition.Mole  y0=[1-env_yO2-env_yH20; env_yO2; 0; env_yH20]  x0=[1; 0; 0; 0]
      settings: InternalSimscapePortConfiguration="{\"Bottom\":[{\"id\":\"H\",\"label\":\"H\",\"type\":\"foundation.thermal.thermal\"}],\"Left\":[{\"id\":\"MIn\",\"label\":\"MIn\",\"type\":\"input\"},{\"id\":\"TIn\",\"label\":\"TIn\",\"type\":\"input\"}],\"Right\":[{\"id\":\"pC\",\"label\":\"p\",\"type\":\"output\"},{\"id\":\"TC\",\"label\":\"T\",\"type\":\"output\"},{\"id\":\"xC_i\",\"label\":\"x_i\",\"type\":\"output\"}],\"Top\":[{\"id\":\"A\",\"label\":\"A\",\"type\":\"FuelCell.FuelCell\"},{\"id\":\"B\",\"label\":\"B\",\"type\":\"FuelCell.FuelCell\"},{\"id\":\"C\",\"label\":\"C\",\"type\":\"FuelCell.FuelCell\"}]}"
  A : PMIOPort  Side=Right
  Min : PMIOPort  Port=2  Side=Right
  Tin : PMIOPort  Port=3  Side=Right
  H : PMIOPort  Port=4  Side=Right
  B : PMIOPort  Port=5  Side=Left
  C : PMIOPort  Port=6  Side=Left
  xi : PMIOPort  Port=7  Side=Left
  connections:
  B/RConn1 -- Cathode/LConn4
  Min/RConn1 -- Cathode/LConn1
  Tin/RConn1 -- Cathode/LConn2
  xi/RConn1 -- Cathode/RConn3
  H/RConn1 -- Cathode/RConn4
  Cathode/LConn5 -- C/RConn1
  A/RConn1 -- Cathode/LConn3

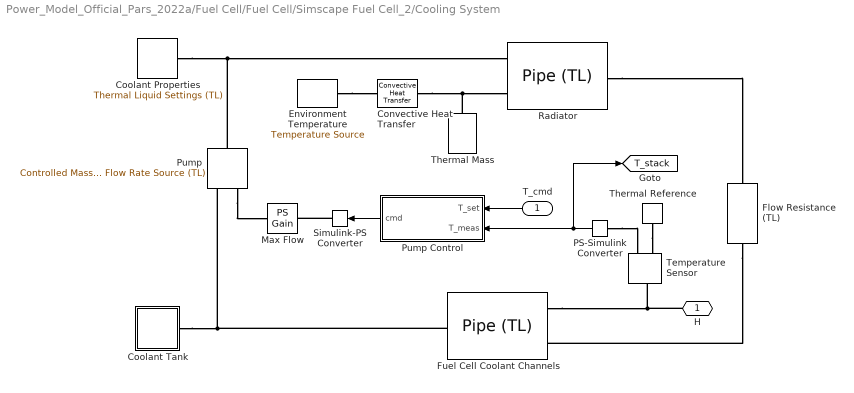
== system Power_Model_Official_Pars_2022a/Fuel Cell/Fuel Cell/Simscape Fuel Cell_2/Cooling System ==
  T_cmd : Inport
  Convective Heat Transfer : fl_lib/Thermal/Thermal Elements/Convective Heat Transfer  thermal_type=foundation.enum.constant_variable.constant  area=radiator_air_area_primary + radiator_eta_fin*radiator_air_area_fins m^2  heat_tr_coeff=300 W/(m^2 * K)  min_heat_tr_coeff=1e-3 W/(K*m^2)  T_specify=off  T_priority=None  T=0 K  T_nominal_specify=off  T_nominal_unit=K  T_nominal_value=1  Q_specify=off  Q_priority=None  Q=0 W  Q_nominal_specify=off  Q_nominal_unit=W  Q_nominal_value=1
  Coolant Properties : fl_lib/Thermal Liquid/Utilities/Thermal Liquid Settings (TL)  table_dimensions=foundation.enum.table_dimensions_TL.two_dimensional  T_TLU=[273.1600 : 10 : 373.16]' K  p_TLU=[0.01, 0.1, 5 : 5 : 50] MPa  p_atm=0.101325 MPa  pT_region_flag=foundation.enum.pT_region_TL.min_max  T_min=273.16 K  T_max=363.16 K  p_min=0.05 MPa  p_max=50 MPa  T_min_1D=273.16 K  T_max_1D=363.16 K  p_min_1D=0.05 MPa  p_max_1D=50 MPa  pT_validity_TLU=[1, 1, 1, 1, 1, 1, 1, 1, 1, 1, 1, 1; 1, 1, 1, 1, 1, 1, 1, 1, 1, 1, 1, 1; 1, 1, 1, 1, 1, 1, 1, 1, 1, 1, 1, 1; 1, 1, 1, 1, 1, 1, 1, 1, 1, 1, 1, 1; 1, 1, 1, 1, 1, 1, 1, 1, 1, 1, 1, 1; 0, 1, 1, 1, 1, 1, 1, 1, 1, 1, 1, 1; 0, 1, 1, 1, 1, 1, 1, 1, 1, 1, 1, 1; 0, 1, 1, 1, 1, 1, 1, 1, 1, 1, 1, 1; 0, 1, 1, 1, 1, 1, 1, 1, 1, 1, 1, 1; 0, 1, 1, 1, 1, 1, 1, 1, 1, 1, 1, 1; 0, 0, 1, 1, 1, 1, 1, 1, 1, 1, 1, 1]  properties_range_check=simscape.enum.assert.action.error  rho_parameterization_2D=foundation.enum.rho_parameterization_2D.rho_beta_alpha  rho_parameterization_1D=foundation.enum.rho_parameterization_1D.rho_vector  rho_TLU=[999.7973, 999.8431, 1002.3216, 1004.8218, 1007.293, 1009.7358, 1012.1506, 1014.5379, 1016.8979, 1019.2311, 1021.538, 1023.8188; 999.6579, 999.7009, 1002.0303, 1004.382, 1006.7084, 1009.0101, 1011.2874, 1013.5407, 1015.7703, 1017.9766, 1020.1599, 1022.3206; 998.1632, 998.2045, 1000.4375, 1002.6924, 1004.9239, 1007.1324, 1009.3183, 1011.4819, 1013.6236, 1015.7438, 1017.8428, 1019.921; 995.6057, 995.6458, 997.81864, 1000.0128, 1002.1841, 1004.3332, 1006.4603, 1008.566, 1010.6505, 1012.7144, 1014.758, 1016.7815; 992.1724, 992.2119, 994.35133, 996.5113, 998.6484, 1000.7633, 1002.8563, 1004.928, 1006.9788, 1009.009, 1011.0192, 1013.0097; 988.02, 988.0299, 990.15684, 992.3035, 994.4268, 996.5273, 998.6056, 1000.6622, 1002.6976, 1004.7123, 1006.7067, 1008.6813; 983.18, 983.1901, 985.3217, 987.4721, 989.5983, 991.7008, 993.7803, 995.8374, 997.8726, 999.8864, 1001.8795, 1003.8522; 977.75, 977.7583, 979.9094, 982.0783, 984.2216, 986.34, 988.4343, 990.505, 992.5529, 994.5786, 996.5825, 998.5654; 971.77, 971.7836, 973.96734, 976.1678, 978.3409, 980.4876, 982.6087, 984.7049, 986.7768, 988.8254, 990.8511, 992.8545; 965.26, 965.3023, 967.53107, 969.7753, 971.9901, 974.1764, 976.3354, 978.4676, 980.5741, 982.6556, 984.7129, 986.7465; 958.62, 958.6315, 960.627, 962.9267, 965.1944, 967.4314, 969.6387, 971.8173, 973.9681, 976.0921, 978.19, 980.2628] kg/m^3  beta_TLU=[1.9649, 1.9654, 1.9929, 2.0213, 2.0499, 2.0787, 2.1078, 2.1372, 2.1668, 2.1966, 2.2268, 2.2572; 2.0913, 2.0918, 2.1191, 2.1471, 2.1752, 2.2036, 2.2322, 2.261, 2.2899, 2.3191, 2.3485, 2.3781; 2.1786, 2.1791, 2.2067, 2.235, 2.2634, 2.2919, 2.3206, 2.3494, 2.3784, 2.4075, 2.4367, 2.4661; 2.2332, 2.2337, 2.2619, 2.2908, 2.3197, 2.3487, 2.3778, 2.407, 2.4363, 2.4657, 2.4951, 2.5246; 2.26, 2.2605, 2.2895, 2.3191, 2.3487, 2.3784, 2.4081, 2.4378, 2.4675, 2.4973, 2.5272, 2.5571; 2.2638, 2.2638, 2.2936, 2.324, 2.3544, 2.3848, 2.4151, 2.4455, 2.4758, 2.5062, 2.5365, 2.5669; 2.2472, 2.2472, 2.2779, 2.3092, 2.3403, 2.3715, 2.4025, 2.4336, 2.4646, 2.4955, 2.5264, 2.5573; 2.214, 2.214, 2.2455, 2.2776, 2.3096, 2.3415, 2.3733, 2.405, 2.4367, 2.4683, 2.4998, 2.5313; 2.1668, 2.1668, 2.1992, 2.2321, 2.2649, 2.2976, 2.3301, 2.3626, 2.3949, 2.4272, 2.4593, 2.4914; 2.1081, 2.1081, 2.1413, 2.175, 2.2086, 2.2421, 2.2754, 2.3085, 2.3415, 2.3744, 2.4072, 2.4399; 2.0494, 2.0494, 2.0739, 2.1084, 2.1428, 2.177, 2.211, 2.2449, 2.2786, 2.3121, 2.3455, 2.3788] GPa  alpha_TLU=1e-4 * [-.679, -.676, -.49, -.307, -.13, .041, .206, .365, .519, .668, .811, .949; .878, .881, .998, 1.114, 1.227, 1.337, 1.445, 1.549, 1.651, 1.75, 1.846, 1.939; 2.068, 2.069, 2.141, 2.213, 2.283, 2.352, 2.42, 2.486, 2.551, 2.614, 2.676, 2.736; 3.034, 3.035, 3.074, 3.113, 3.152, 3.191, 3.229, 3.267, 3.305, 3.341, 3.377, 3.413; 3.855, 3.856, 3.87, 3.884, 3.899, 3.914, 3.93, 3.946, 3.961, 3.977, 3.993, 4.009; 4.578, 4.578, 4.572, 4.566, 4.562, 4.558, 4.555, 4.552, 4.55, 4.549, 4.548, 4.547; 5.233, 5.233, 5.209, 5.186, 5.165, 5.144, 5.125, 5.107, 5.09, 5.074, 5.059, 5.045; 5.84, 5.84, 5.801, 5.762, 5.725, 5.691, 5.657, 5.625, 5.595, 5.566, 5.538, 5.512; 6.414, 6.414, 6.36, 6.307, 6.256, 6.208, 6.161, 6.117, 6.074, 6.033, 5.994, 5.956; 6.967, 6.967, 6.898, 6.831, 6.766, 6.705, 6.646, 6.589, 6.535, 6.482, 6.432, 6.384; 7.519, 7.519, 7.423, 7.342, 7.264, 7.189, 7.118, 7.049, 6.983, 6.92, 6.859, 6.8] 1/K  rho_TLU_2=[999.7973, 999.8431, 1002.3216, 1004.8218, 1007.293, 1009.7358, 1012.1506, 1014.5379, 1016.8979, 1019.2311, 1021.538, 1023.8188; 999.6579, 999.7009, 1002.0303, 1004.382, 1006.7084, 1009.0101, 1011.2874, 1013.5407, 1015.7703, 1017.9766, 1020.1599, 1022.3206; 998.1632, 998.2045, 1000.4375, 1002.6924, 1004.9239, 1007.1324, 1009.3183, 1011.4819, 1013.6236, 1015.7438, 1017.8428, 1019.921; 995.6057, 995.6458, 997.81864, 1000.0128, 1002.1841, 1004.3332, 1006.4603, 1008.566, 1010.6505, 1012.7144, 1014.758, 1016.7815; 992.1724, 992.2119, 994.35133, 996.5113, 998.6484, 1000.7633, 1002.8563, 1004.928, 1006.9788, 1009.009, 1011.0192, 1013.0097; 988.02, 988.0299, 990.15684, 992.3035, 994.4268, 996.5273, 998.6056, 1000.6622, 1002.6976, 1004.7123, 1006.7067, 1008.6813; 983.18, 983.1901, 985.3217, 987.4721, 989.5983, 991.7008, 993.7803, 995.8374, 997.8726, 999.8864, 1001.8795, 1003.8522; 977.75, 977.7583, 979.9094, 982.0783, 984.2216, 986.34, 988.4343, 990.505, 992.5529, 994.5786, 996.5825, 998.5654; 971.77, 971.7836, 973.96734, 976.1678, 978.3409, 980.4876, 982.6087, 984.7049, 986.7768, 988.8254, 990.8511, 992.8545; 965.26, 965.3023, 967.53107, 969.7753, 971.9901, 974.1764, 976.3354, 978.4676, 980.5741, 982.6556, 984.7129, 986.7465; 958.62, 958.6315, 960.627, 962.9267, 965.1944, 967.4314, 969.6387, 971.8173, 973.9681, 976.0921, 978.19, 980.2628] kg/m^3  rho_ref_3=998.21 kg/m^3  T_ref_3=293.16 K  p_ref_3=0.101325 MPa  beta_const_3=2.1791 GPa  alpha_const_3=2.0691e-4 1/K  rho_TLU_4=[999.84; 999.7; 998.2; 995.65; 992.21; 988.03; 983.19; 977.76; 971.78; 965.3; 958.8] kg/m^3  beta_const_4=2.1791 GPa  p_ref_4=0.101325 MPa  rho_ref_5=998.21 kg/m^3  T_ref_5=293.16 K  p_ref_5=0.101325 MPa  beta_const_5=2.1791 GPa  alpha_const_5=2.0691e-4 1/K  u_parameterization_2D=foundation.enum.u_parameterization_2D.u_cp  u_parameterization_1D=foundation.enum.u_parameterization_1D.u  u_TLU=[.0002, .0018, .086, .1588, .219, .267, .3034, .3288, .3436, .3483, .3435, .3294; 42.062, 42.06, 41.935, 41.804, 41.668, 41.527, 41.382, 41.233, 41.081, 40.924, 40.763, 40.599; 83.953, 83.948, 83.651, 83.349, 83.049, 82.749, 82.451, 82.153, 81.856, 81.56, 81.265, 80.971; 125.77, 125.76, 125.31, 124.86, 124.41, 123.97, 123.53, 123.1, 122.68, 122.25, 121.84, 121.42; 167.57, 167.56, 166.96, 166.37, 165.79, 165.21, 164.65, 164.09, 163.54, 163, 162.46, 161.94; 209.36, 209.36, 208.63, 207.9, 207.19, 206.48, 205.79, 205.11, 204.45, 203.79, 203.14, 202.5; 251.19, 251.19, 250.33, 249.47, 248.62, 247.79, 246.98, 246.18, 245.39, 244.62, 243.86, 243.12; 293.06, 293.06, 292.07, 291.07, 290.1, 289.14, 288.2, 287.28, 286.38, 285.49, 284.62, 283.77; 334.99, 334.99, 333.86, 332.73, 331.63, 330.54, 329.48, 328.44, 327.41, 326.41, 325.43, 324.46; 377, 377, 375.73, 374.46, 373.22, 372, 370.81, 369.64, 368.5, 367.38, 366.27, 365.19; 419.01, 419.01, 417.69, 416.27, 414.89, 413.54, 412.21, 410.91, 409.64, 408.4, 407.17, 405.98] kJ/kg  cp_TLU=[4.2199, 4.2194, 4.1957, 4.1726, 4.1508, 4.13, 4.1103, 4.0916, 4.0738, 4.0569, 4.0408, 4.0254; 4.1955, 4.1951, 4.1769, 4.1592, 4.1422, 4.1259, 4.1103, 4.0954, 4.0812, 4.0676, 4.0545, 4.0421; 4.1843, 4.184, 4.169, 4.1543, 4.1401, 4.1264, 4.1133, 4.1007, 4.0885, 4.0768, 4.0656, 4.0548; 4.1801, 4.1798, 4.1667, 4.1538, 4.1413, 4.1293, 4.1177, 4.1064, 4.0956, 4.0851, 4.075, 4.0653; 4.1796, 4.1794, 4.1675, 4.1558, 4.1444, 4.1334, 4.1227, 4.1123, 4.1023, 4.0926, 4.0832, 4.0741; 4.1813, 4.1813, 4.1702, 4.1592, 4.1484, 4.138, 4.1279, 4.1181, 4.1086, 4.0993, 4.0903, 4.0816; 4.185, 4.185, 4.1742, 4.1636, 4.1532, 4.1432, 4.1334, 4.1239, 4.1146, 4.1056, 4.0969, 4.0884; 4.1901, 4.1901, 4.1795, 4.169, 4.1588, 4.1489, 4.1393, 4.1299, 4.1207, 4.1118, 4.1032, 4.0947; 4.1968, 4.1968, 4.1862, 4.1757, 4.1655, 4.1555, 4.1458, 4.1364, 4.1273, 4.1183, 4.1096, 4.1012; 4.2052, 4.2052, 4.1944, 4.1837, 4.1733, 4.1632, 4.1534, 4.1438, 4.1345, 4.1255, 4.1166, 4.108; 4.2136, 4.2136, 4.2045, 4.1935, 4.1828, 4.1724, 4.1623, 4.1524, 4.1429, 4.1335, 4.1245, 4.1157] kJ/kg/K  u_TLU_2=[.0002, .0018, .086, .1588, .219, .267, .3034, .3288, .3436, .3483, .3435, .3294; 42.062, 42.06, 41.935, 41.804, 41.668, 41.527, 41.382, 41.233, 41.081, 40.924, 40.763, 40.599; 83.953, 83.948, 83.651, 83.349, 83.049, 82.749, 82.451, 82.153, 81.856, 81.56, 81.265, 80.971; 125.77, 125.76, 125.31, 124.86, 124.41, 123.97, 123.53, 123.1, 122.68, 122.25, 121.84, 121.42; 167.57, 167.56, 166.96, 166.37, 165.79, 165.21, 164.65, 164.09, 163.54, 163, 162.46, 161.94; 209.36, 209.36, 208.63, 207.9, 207.19, 206.48, 205.79, 205.11, 204.45, 203.79, 203.14, 202.5; 251.19, 251.19, 250.33, 249.47, 248.62, 247.79, 246.98, 246.18, 245.39, 244.62, 243.86, 243.12; 293.06, 293.06, 292.07, 291.07, 290.1, 289.14, 288.2, 287.28, 286.38, 285.49, 284.62, 283.77; 334.99, 334.99, 333.86, 332.73, 331.63, 330.54, 329.48, 328.44, 327.41, 326.41, 325.43, 324.46; 377, 377, 375.73, 374.46, 373.22, 372, 370.81, 369.64, 368.5, 367.38, 366.27, 365.19; 419.01, 419.01, 417.69, 416.27, 414.89, 413.54, 412.21, 410.91, 409.64, 408.4, 407.17, 405.98] kJ/kg  cp_TLU_3=[4.2199, 4.2194, 4.1957, 4.1726, 4.1508, 4.13, 4.1103, 4.0916, 4.0738, 4.0569, 4.0408, 4.0254; 4.1955, 4.1951, 4.1769, 4.1592, 4.1422, 4.1259, 4.1103, 4.0954, 4.0812, 4.0676, 4.0545, 4.0421; 4.1843, 4.184, 4.169, 4.1543, 4.1401, 4.1264, 4.1133, 4.1007, 4.0885, 4.0768, 4.0656, 4.0548; 4.1801, 4.1798, 4.1667, 4.1538, 4.1413, 4.1293, 4.1177, 4.1064, 4.0956, 4.0851, 4.075, 4.0653; 4.1796, 4.1794, 4.1675, 4.1558, 4.1444, 4.1334, 4.1227, 4.1123, 4.1023, 4.0926, 4.0832, 4.0741; 4.1813, 4.1813, 4.1702, 4.1592, 4.1484, 4.138, 4.1279, 4.1181, 4.1086, 4.0993, 4.0903, 4.0816; 4.185, 4.185, 4.1742, 4.1636, 4.1532, 4.1432, 4.1334, 4.1239, 4.1146, 4.1056, 4.0969, 4.0884; 4.1901, 4.1901, 4.1795, 4.169, 4.1588, 4.1489, 4.1393, 4.1299, 4.1207, 4.1118, 4.1032, 4.0947; 4.1968, 4.1968, 4.1862, 4.1757, 4.1655, 4.1555, 4.1458, 4.1364, 4.1273, 4.1183, 4.1096, 4.1012; 4.2052, 4.2052, 4.1944, 4.1837, 4.1733, 4.1632, 4.1534, 4.1438, 4.1345, 4.1255, 4.1166, 4.108; 4.2136, 4.2136, 4.2045, 4.1935, 4.1828, 4.1724, 4.1623, 4.1524, 4.1429, 4.1335, 4.1245, 4.1157] kJ/kg/K  u_TLU_4=[.0018; 42.06; 83.948; 125.76; 167.56; 209.36; 251.19; 293.06; 334.99; 377; 418.01] kJ/kg  cp_TLU_5=[4.2199; 4.1955; 4.1843; 4.1801; 4.1796; 4.1813; 4.185; 4.1901; 4.1968; 4.2052; 4.2136] kJ/kg/K  nu_TLU=[1.7917, 1.7914, 1.7763, 1.7615, 1.7473, 1.7338, 1.7208, 1.7085, 1.6967, 1.6854, 1.6747, 1.6645; 1.3061, 1.3059, 1.2986, 1.2914, 1.2845, 1.2779, 1.2716, 1.2656, 1.2598, 1.2543, 1.2491, 1.2441; 1.0032, 1.0032, .9995, .9959, .9924, .9891, .9859, .9829, .9801, .9774, .9748, .9724; .8006, .8005, .7987, .797, .7953, .7937, .7922, .7908, .7894, .7881, .787, .7859; .6577, .6577, .657, .6562, .6555, .6548, .6543, .6537, .6532, .6528, .6523, .652; .553, .553, .5529, .5527, .5526, .5525, .5524, .5524, .5524, .5524, .5524, .5525; .4739, .4739, .4741, .4743, .4745, .4747, .475, .4753, .4755, .4758, .4762, .4765; .4127, .4127, .4131, .4135, .4139, .4143, .4148, .4152, .4157, .4162, .4167, .4172; .3643, .3643, .3648, .3654, .3659, .3665, .367, .3676, .3682, .3688, .3694, .37; .3254, .3254, .3261, .3267, .3273, .328, .3286, .3293, .3299, .3306, .3312, .3319; .2866, .2866, .2945, .2952, .2959, .2965, .2972, .2979, .2986, .2993, .3, .3007] mm^2/s  nu_TLU_2=[1.7917; 1.3061; 1.0032; .8006; .6577; .553; .4739; .4127; .3643; .3254; .2866] mm^2/s  k_TLU=[561.04, 561.09, 563.8, 566.56, 569.32, 572.08, 574.82, 577.54, 580.24, 582.92, 585.57, 588.18; 580.02, 580.07, 582.45, 584.88, 587.32, 589.75, 592.18, 594.61, 597.02, 599.42, 601.8, 604.16; 598.44, 598.48, 600.73, 603.03, 605.33, 607.64, 609.94, 612.24, 614.54, 616.82, 619.1, 621.36; 615.48, 615.52, 617.73, 620, 622.26, 624.54, 626.81, 629.07, 631.34, 633.6, 635.85, 638.09; 630.6, 630.64, 632.87, 635.15, 637.44, 639.72, 642.01, 644.29, 646.57, 648.84, 651.11, 653.36; 643.61, 643.61, 645.88, 648.21, 650.53, 652.86, 655.18, 657.51, 659.82, 662.14, 664.44, 666.74; 654.39, 654.39, 656.73, 659.12, 661.5, 663.89, 666.27, 668.65, 671.02, 673.38, 675.74, 678.09; 663.13, 663.13, 665.54, 668, 670.46, 672.91, 675.36, 677.8, 680.24, 682.67, 685.09, 687.5; 670.02, 670.02, 672.51, 675.05, 677.59, 680.12, 682.64, 685.16, 687.67, 690.17, 692.66, 695.14; 675.27, 675.27, 677.85, 680.48, 683.11, 685.73, 688.34, 690.94, 693.53, 696.11, 698.68, 701.24; 680.52, 680.52, 681.77, 684.5, 687.22, 689.94, 692.64, 695.34, 698.02, 700.69, 703.35, 706] mW/m/K  k_TLU_2=[561.04; 580.02; 598.44; 615.48; 630.6; 643.61; 654.39; 663.13; 670.02; 675.27; 680.52] mW/m/K
  Coolant Tank : Subsystem  Tag=PublishSubsystem  mask(Coolant Tank){A=0.1, x_init=0.08}
      mask prompts: A "Tank area (m^2)"; x_init "Initial coolant level (m)"
      mask help: This subsystem models an expansion tank for the coolant system.
  Environment Temperature : fl_lib/Thermal/Thermal Sources/Temperature Source  temperature=env_T degC
  Flow Resistance (TL) : fl_lib/Thermal Liquid/Elements/Flow Resistance (TL)  delta_p_nominal=0.001 MPa  mdot_nominal=0.1 kg/s  area=pi*coolant_tube_D^2/4 m^2  laminar_fraction=1e-3
  Fuel Cell Coolant Channels : fl_lib/Thermal Liquid/Elements/Pipe (TL)  length=sqrt(stack_area) * coolant_num_passes cm  area=coolant_w_channels^2 * coolant_num_layers cm^2  Dh=coolant_w_channels cm  length_add=10 cm  roughness=15e-6 m  Re_lam=2000  Re_tur=4000  shape_factor=64  Nu_lam=3.66  dynamic_compressibility=simscape.enum.onoff.on  inertia=simscape.enum.onoff.off  p0=env_p MPa  T0=env_T degC  mdot0=0 kg/s
  Max Flow : fl_lib/Physical Signals/Functions/PS Gain  gain=2 kg/s
  PS-Simulink Converter : nesl_utility/PS-Simulink Converter  PhysicalDomain=network_engine_domain  SubClassName=ps_output  LeftPortType=input  RightPortType=output  PseudoPeriodic=off  Frequencies=[]  VectorFormat=1-D array  Unit=degC  AffineConversion=on
  Pump : fl_lib/Thermal Liquid/Sources/Controlled Mass Flow Rate Source (TL)  power_spec=foundation.enum.power_spec.isentropic  area=pi*coolant_tube_D^2/4 m^2
      settings: InternalSimscapePortConfiguration="{\"Bottom\":[],\"Left\":[{\"id\":\"A\",\"label\":\"A\",\"type\":\"foundation.thermal_liquid.thermal_liquid\"},{\"id\":\"M\",\"label\":\"M\",\"type\":\"input\"}],\"Right\":[{\"id\":\"B\",\"label\":\"B\",\"type\":\"foundation.thermal_liquid.thermal_liquid\"}],\"Top\":[]}"
  Pump Control : Subsystem
  Radiator : fl_lib/Thermal Liquid/Elements/Pipe (TL)  length=radiator_L m  area=radiator_W * radiator_tube_H * radiator_N_tubes m^2  Dh=2*radiator_W*radiator_tube_H / (radiator_W + radiator_tube_H) m  length_add=radiator_tube_Leq m  roughness=15e-6 m  Re_lam=2000  Re_tur=4000  shape_factor=64  Nu_lam=3.66  dynamic_compressibility=simscape.enum.onoff.on  inertia=simscape.enum.onoff.off  p0=env_p MPa  T0=env_T degC  mdot0=0 kg/s
  Simulink-PS Converter : nesl_utility/Simulink-PS Converter  PhysicalDomain=network_engine_domain  SubClassName=ps_input  LeftPortType=input  RightPortType=output  PseudoPeriodic=off  Frequencies=[]  NoiseDistribution=none  NoiseParameters=[]  Unit=1  AffineConversion=off  FilteringAndDerivatives=provide  SimscapeFilterOrder=1  InputFilterTimeConstant=0.001  UdotUserProvided=0
  Temperature Sensor : fl_lib/Thermal/Thermal Sensors/Temperature Sensor  temperature_measure=foundation.enum.MeasurementReference.difference
  Thermal Mass : fl_lib/Thermal/Thermal Elements/Thermal Mass  mass_type=foundation.enum.constant_variable.constant  mass=(radiator_air_area_primary + radiator_air_area_fins) * radiator_t_wall * radiator_rho kg  sp_heat=radiator_cp J/kg/K  mass_min=1e-6 kg  num_ports=foundation.enum.numPorts2.one  m_specify=off  m_priority=High  m=1 kg  m_nominal_specify=off  m_nominal_unit=kg  m_nominal_value=1  T_specify=on  T_priority=High  T=env_T degC  T_nominal_specify=off  T_nominal_unit=K  T_nominal_value=1  Q_specify=off  Q_priority=None  Q=0 W  Q_nominal_specify=off  Q_nominal_unit=W  Q_nominal_value=1
  Thermal Reference : fl_lib/Thermal/Thermal Elements/Thermal Reference
  H : PMIOPort  Side=Right
  tag scope: T_stack=global
  wires:
  Pump Control/1(cmd) -> Simulink-PS Converter/1
  PS-Simulink Converter/1 -> Pump Control/2(T_meas), [T_stack]
  T_cmd/1 -> Pump Control/1(T_set)
  connections:
  Pump/RConn1 -- Radiator/LConn1 -- Coolant Properties/RConn1
  Fuel Cell Coolant Channels/RConn1 -- Coolant Tank/RConn1 -- Pump/LConn1
  Convective Heat Transfer/LConn1 -- Thermal Mass/LConn1 -- Radiator/LConn2
  Environment Temperature/LConn1 -- Convective Heat Transfer/RConn1
  Thermal Reference/LConn1 -- Temperature Sensor/RConn1
  Radiator/RConn1 -- Flow Resistance (TL)/LConn1
  PS-Simulink Converter/LConn1 -- Temperature Sensor/RConn2
  Pump/LConn2 -- Max Flow/RConn1
  Simulink-PS Converter/RConn1 -- Max Flow/LConn1
  Flow Resistance (TL)/RConn1 -- Fuel Cell Coolant Channels/LConn1
  H/RConn1 -- Temperature Sensor/LConn1 -- Fuel Cell Coolant Channels/LConn2

== system Power_Model_Official_Pars_2022a/Fuel Cell/Fuel Cell/Simscape Fuel Cell_2/Heat Dissipation ==
  Heat Flow Rate Sensor : fl_lib/Thermal/Thermal Sensors/Heat Flow Rate Sensor
  PS-Simulink Converter : nesl_utility/PS-Simulink Converter  PhysicalDomain=network_engine_domain  SubClassName=ps_output  LeftPortType=input  RightPortType=output  PseudoPeriodic=off  Frequencies=[]  VectorFormat=1-D array  Unit=kW  AffineConversion=off
  A : PMIOPort  Side=Left
  B : PMIOPort  Port=2  Side=Right
  tag scope: Q_stack=global
  wires:
  PS-Simulink Converter/1 -> [Q_stack]
  connections:
  A/RConn1 -- Heat Flow Rate Sensor/LConn1
  B/RConn1 -- Heat Flow Rate Sensor/RConn2
  Heat Flow Rate Sensor/RConn1 -- PS-Simulink Converter/LConn1
